simulink model "vector_control"  (R2020a)
settings: Solver=ode23t  StartTime=0.0  StopTime=2  RelTol=1e-3
libraries: powerlib x22, powerlib_meascontrol x6, simulink x4
settings Model: Creator=ahmed  LastModifiedBy=ahmed

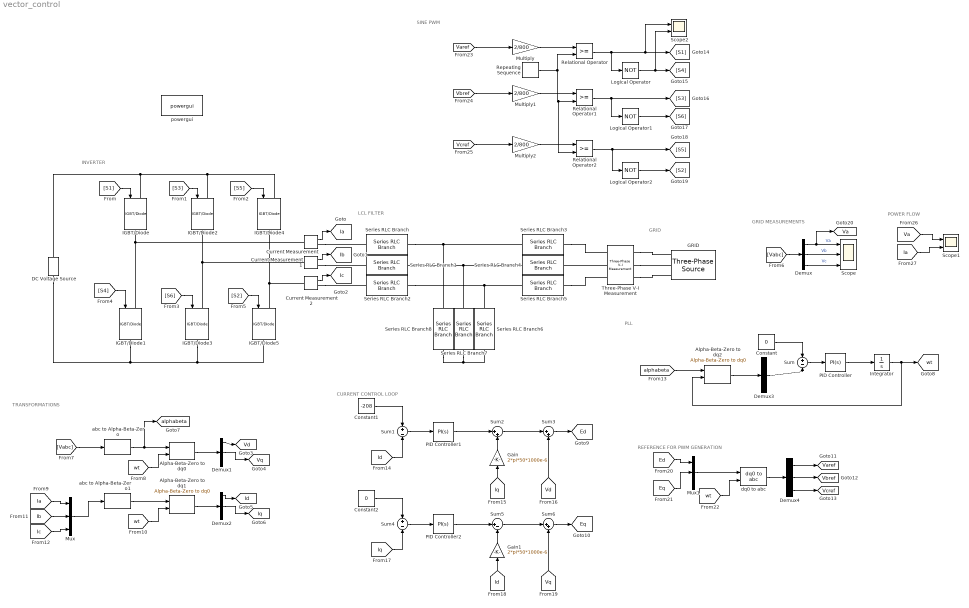
== system vector_control ==
  note: POWER FLOW
  note: GRID MEASUREMENTS
  note: GRID
  note: TRANSFORMATIONS
  note: CURRENT CONTROL LOOP
  note: REFERENCE FOR PWM GENERATION
  note: PLL
  note: SINE PWM
  note: LCL FILTER
  note: INVERTER
  Alpha-Beta-Zero to dq0 : powerlib_meascontrol/Transformations/Alpha-Beta-Zero to dq0  Alignment=90 degrees behind phase A axis
  Alpha-Beta-Zero to dq1 : powerlib_meascontrol/Transformations/Alpha-Beta-Zero to dq0  Alignment=90 degrees behind phase A axis
  Alpha-Beta-Zero to dq2 : powerlib_meascontrol/Transformations/Alpha-Beta-Zero to dq0  Alignment=90 degrees behind phase A axis
  Constant : Constant  Value=0
  Constant1 : Constant  Value=-208
  Constant2 : Constant  Value=0
  Current Measurement : powerlib/Measurements/Current Measurement  PhasorSimulation=off  OutputType=Complex  PSBequivalent=0
  Current Measurement1 : powerlib/Measurements/Current Measurement  PhasorSimulation=off  OutputType=Complex  PSBequivalent=0
  Current Measurement2 : powerlib/Measurements/Current Measurement  PhasorSimulation=off  OutputType=Complex  PSBequivalent=0
  DC Voltage Source : powerlib/Electrical Sources/DC Voltage Source  Amplitude=800  Measurements=None
  Demux{,1..4} (5 alike) : Demux  Outputs=3
  GRID : powerlib/Electrical Sources/Three-Phase Source  InternalConnection=Yg  VoltagePhases=off  Voltage=415  PhaseAngle=0  Voltage_phases=[25e3 25e3 25e3]/sqrt(3)  PhaseAngles_phases=[0 -120 +120]  Frequency=50  NonIdealSource=on  SpecifyImpedance=off  Resistance=0.001e-3  Inductance=0.001e-9  ShortCircuitLevel=100e6  BaseVoltage=415  XRratio=7  BusType=swing  Pref=10e3  Qref=0  Prefabc=[10e3, 10e3, 10e3]  Qrefabc=[0, 0, 0]  Qmin=-inf  Qmax=inf
  Gain : Gain  Gain=2*pi*50*1000e-6
  Gain1 : Gain  Gain=2*pi*50*1000e-6
  IGBT/Diode{,1..5} (6 alike) : powerlib/Power Electronics/IGBT//Diode  Ron=1e-3  Rs=1e5  Cs=inf  Measurements=off
  Integrator : Integrator
  Logical Operator : Logic  Operator=NOT  AllPortsSameDT=off  OutDataTypeStr=boolean
  Logical Operator1 : Logic  Operator=NOT  AllPortsSameDT=off  OutDataTypeStr=boolean
  Logical Operator2 : Logic  Operator=NOT  AllPortsSameDT=off  OutDataTypeStr=boolean
  Multiply : Gain  Gain=2/800
  Multiply1 : Gain  Gain=2/800
  Multiply2 : Gain  Gain=2/800
  Mux : Mux  Inputs=3
  Mux1 : Mux  Inputs=3
  PID Controller : simulink/Continuous/PID Controller  Controller=PI  Form=Parallel  TimeDomain=Continuous-time  UseExternalTs=off  SampleTime=-1  IntegratorMethod=Forward Euler  FilterMethod=Forward Euler  ControllerParametersSource=internal  P=10  I=50000  D=0  UseFilter=on  N=100  TunerSelectOption=Transfer Function Based (PID Tuner App)  InitialConditionSource=internal  InitialConditionForIntegrator=0  InitialConditionForFilter=0  DifferentiatorICPrevScaledInput=0  ExternalReset=none  TrackingMode=off  Kt=1  LimitOutput=off  UpperSaturationLimit=inf  LowerSaturationLimit=-inf  LinearizeAsGain=on  AntiWindupMode=none  Kb=1  POutMin=[]  POutMax=[]  IOutMin=[]  IOutMax=[]  DOutMin=[]  DOutMax=[]  NOutMin=[]  NOutMax=[]  SumOutMin=[]  SumOutMax=[]  SaturationOutMin=[]  SaturationOutMax=[]  PParamMin=[]  PParamMax=[]  IParamMin=[]  IParamMax=[]  DParamMin=[]  DParamMax=[]  NParamMin=[]  NParamMax=[]  KbParamMin=[]  KbParamMax=[]  KtParamMin=[]  KtParamMax=[]  KbOutMin=[]  KbOutMax=[]  KtOutMin=[]  KtOutMax=[]  IntegratorOutMin=[]  IntegratorOutMax=[]  FilterOutMin=[]  FilterOutMax=[]  SumI1OutMin=[]  SumI1OutMax=[]  SumI2OutMin=[]  SumI2OutMax=[]  SumI3OutMin=[]  SumI3OutMax=[]  SumI4OutMin=[]  SumI4OutMax=[]  SumDOutMin=[]  SumDOutMax=[]  DifferentiatorOutMin=[]  DifferentiatorOutMax=[]  FilterDiffOutCoefMin=[]  FilterDiffOutCoefMax=[]  ReciprocalOutMin=[]  ReciprocalOutMax=[]  SumDenOutMin=[]  SumDenOutMax=[]  SumNumOutMin=[]  SumNumOutMax=[]  DivideOutMin=[]  DivideOutMax=[]  UdiffTsProdOutMin=[]  UdiffTsProdOutMax=[]  NTsProdOutMin=[]  NTsProdOutMax=[]  UintegralTsProdOutMin=[]  UintegralTsProdOutMax=[]  UngainTsProdOutMin=[]  UngainTsProdOutMax=[]  IntegratorContinuousStateAttributes=''  IntegratorStateMustResolveToSignalObject=off  IntegratorRTWStateStorageClass=Auto  FilterContinuousStateAttributes=''  FilterStateMustResolveToSignalObject=off  FilterRTWStateStorageClass=Auto  ParallelPVariant=InternalParameters  IdealPVariant=Disabled  IVariant=InternalParameters  DVariant=Disabled  IntegratorVariant=Continuous  SatVariant=Disabled  AWVariant=Passthrough  PCopyVariant=Disabled  TRVariant=Disabled  FdbkBlocksVariant=Forward  IdealPFdbkVariant=Disabled  SatFdbkVariant=Disabled  DerivativeFilterVariant=Disabled  NVariant=Disabled  NCopyVariant=Disabled_SignalSpec  FilterICVariant=Disabled  IntegratorICVariant=InternalICs  ExternalResetVariant=Disabled  TRSumVariant=Passthrough  SumFdbkVariant=Disabled  SumVariant=Sum_PI  TsampFilterVariant=InternalTs  TsampNgainVariant=Passthrough  TsampIntegralVariant=Passthrough
  PID Controller1 : simulink/Continuous/PID Controller  Controller=PI  Form=Parallel  TimeDomain=Continuous-time  UseExternalTs=off  SampleTime=-1  IntegratorMethod=Forward Euler  FilterMethod=Forward Euler  ControllerParametersSource=internal  P=5  I=5000  D=0  UseFilter=on  N=100  TunerSelectOption=Transfer Function Based (PID Tuner App)  InitialConditionSource=internal  InitialConditionForIntegrator=0  InitialConditionForFilter=0  DifferentiatorICPrevScaledInput=0  ExternalReset=none  TrackingMode=off  Kt=1  LimitOutput=off  UpperSaturationLimit=inf  LowerSaturationLimit=-inf  LinearizeAsGain=on  AntiWindupMode=none  Kb=1  POutMin=[]  POutMax=[]  IOutMin=[]  IOutMax=[]  DOutMin=[]  DOutMax=[]  NOutMin=[]  NOutMax=[]  SumOutMin=[]  SumOutMax=[]  SaturationOutMin=[]  SaturationOutMax=[]  PParamMin=[]  PParamMax=[]  IParamMin=[]  IParamMax=[]  DParamMin=[]  DParamMax=[]  NParamMin=[]  NParamMax=[]  KbParamMin=[]  KbParamMax=[]  KtParamMin=[]  KtParamMax=[]  KbOutMin=[]  KbOutMax=[]  KtOutMin=[]  KtOutMax=[]  IntegratorOutMin=[]  IntegratorOutMax=[]  FilterOutMin=[]  FilterOutMax=[]  SumI1OutMin=[]  SumI1OutMax=[]  SumI2OutMin=[]  SumI2OutMax=[]  SumI3OutMin=[]  SumI3OutMax=[]  SumI4OutMin=[]  SumI4OutMax=[]  SumDOutMin=[]  SumDOutMax=[]  DifferentiatorOutMin=[]  DifferentiatorOutMax=[]  FilterDiffOutCoefMin=[]  FilterDiffOutCoefMax=[]  ReciprocalOutMin=[]  ReciprocalOutMax=[]  SumDenOutMin=[]  SumDenOutMax=[]  SumNumOutMin=[]  SumNumOutMax=[]  DivideOutMin=[]  DivideOutMax=[]  UdiffTsProdOutMin=[]  UdiffTsProdOutMax=[]  NTsProdOutMin=[]  NTsProdOutMax=[]  UintegralTsProdOutMin=[]  UintegralTsProdOutMax=[]  UngainTsProdOutMin=[]  UngainTsProdOutMax=[]  IntegratorContinuousStateAttributes=''  IntegratorStateMustResolveToSignalObject=off  IntegratorRTWStateStorageClass=Auto  FilterContinuousStateAttributes=''  FilterStateMustResolveToSignalObject=off  FilterRTWStateStorageClass=Auto  ParallelPVariant=InternalParameters  IdealPVariant=Disabled  IVariant=InternalParameters  DVariant=Disabled  IntegratorVariant=Continuous  SatVariant=Disabled  AWVariant=Passthrough  PCopyVariant=Disabled  TRVariant=Disabled  FdbkBlocksVariant=Forward  IdealPFdbkVariant=Disabled  SatFdbkVariant=Disabled  DerivativeFilterVariant=Disabled  NVariant=Disabled  NCopyVariant=Disabled_SignalSpec  FilterICVariant=Disabled  IntegratorICVariant=InternalICs  ExternalResetVariant=Disabled  TRSumVariant=Passthrough  SumFdbkVariant=Disabled  SumVariant=Sum_PI  TsampFilterVariant=InternalTs  TsampNgainVariant=Passthrough  TsampIntegralVariant=Passthrough
  PID Controller2 : simulink/Continuous/PID Controller  Controller=PI  Form=Parallel  TimeDomain=Continuous-time  UseExternalTs=off  SampleTime=-1  IntegratorMethod=Forward Euler  FilterMethod=Forward Euler  ControllerParametersSource=internal  P=5  I=5000  D=0  UseFilter=on  N=100  TunerSelectOption=Transfer Function Based (PID Tuner App)  InitialConditionSource=internal  InitialConditionForIntegrator=0  InitialConditionForFilter=0  DifferentiatorICPrevScaledInput=0  ExternalReset=none  TrackingMode=off  Kt=1  LimitOutput=off  UpperSaturationLimit=inf  LowerSaturationLimit=-inf  LinearizeAsGain=on  AntiWindupMode=none  Kb=1  POutMin=[]  POutMax=[]  IOutMin=[]  IOutMax=[]  DOutMin=[]  DOutMax=[]  NOutMin=[]  NOutMax=[]  SumOutMin=[]  SumOutMax=[]  SaturationOutMin=[]  SaturationOutMax=[]  PParamMin=[]  PParamMax=[]  IParamMin=[]  IParamMax=[]  DParamMin=[]  DParamMax=[]  NParamMin=[]  NParamMax=[]  KbParamMin=[]  KbParamMax=[]  KtParamMin=[]  KtParamMax=[]  KbOutMin=[]  KbOutMax=[]  KtOutMin=[]  KtOutMax=[]  IntegratorOutMin=[]  IntegratorOutMax=[]  FilterOutMin=[]  FilterOutMax=[]  SumI1OutMin=[]  SumI1OutMax=[]  SumI2OutMin=[]  SumI2OutMax=[]  SumI3OutMin=[]  SumI3OutMax=[]  SumI4OutMin=[]  SumI4OutMax=[]  SumDOutMin=[]  SumDOutMax=[]  DifferentiatorOutMin=[]  DifferentiatorOutMax=[]  FilterDiffOutCoefMin=[]  FilterDiffOutCoefMax=[]  ReciprocalOutMin=[]  ReciprocalOutMax=[]  SumDenOutMin=[]  SumDenOutMax=[]  SumNumOutMin=[]  SumNumOutMax=[]  DivideOutMin=[]  DivideOutMax=[]  UdiffTsProdOutMin=[]  UdiffTsProdOutMax=[]  NTsProdOutMin=[]  NTsProdOutMax=[]  UintegralTsProdOutMin=[]  UintegralTsProdOutMax=[]  UngainTsProdOutMin=[]  UngainTsProdOutMax=[]  IntegratorContinuousStateAttributes=''  IntegratorStateMustResolveToSignalObject=off  IntegratorRTWStateStorageClass=Auto  FilterContinuousStateAttributes=''  FilterStateMustResolveToSignalObject=off  FilterRTWStateStorageClass=Auto  ParallelPVariant=InternalParameters  IdealPVariant=Disabled  IVariant=InternalParameters  DVariant=Disabled  IntegratorVariant=Continuous  SatVariant=Disabled  AWVariant=Passthrough  PCopyVariant=Disabled  TRVariant=Disabled  FdbkBlocksVariant=Forward  IdealPFdbkVariant=Disabled  SatFdbkVariant=Disabled  DerivativeFilterVariant=Disabled  NVariant=Disabled  NCopyVariant=Disabled_SignalSpec  FilterICVariant=Disabled  IntegratorICVariant=InternalICs  ExternalResetVariant=Disabled  TRSumVariant=Passthrough  SumFdbkVariant=Disabled  SumVariant=Sum_PI  TsampFilterVariant=InternalTs  TsampNgainVariant=Passthrough  TsampIntegralVariant=Passthrough
  Relational Operator : RelationalOperator  OutDataTypeStr=boolean  RndMeth=Simplest
  Relational Operator1 : RelationalOperator  OutDataTypeStr=boolean  RndMeth=Simplest
  Relational Operator2 : RelationalOperator  OutDataTypeStr=boolean  RndMeth=Simplest
  Repeating Sequence : simulink/Sources/Repeating Sequence  rep_seq_t=[0 0.00005 0.0001]  rep_seq_y=[-1 1 -1]
  Scope : Scope  NumInputPorts=3
  Scope1 : Scope  NumInputPorts=2
  Scope2 : Scope  NumInputPorts=2
  Series RLC Branch{,1..5} (6 alike) : powerlib/Elements/Series RLC Branch  LConnTagsString=__new0  RConnTagsString=__new0  BranchType=L  Resistance=1  Inductance=500e-6  SetiL0=off  InitialCurrent=0  Capacitance=1e-6  Setx0=off  InitialVoltage=0  Measurements=None
  Series RLC Branch6 : powerlib/Elements/Series RLC Branch  LConnTagsString=__new0  RConnTagsString=__new0  BranchType=L  Resistance=1  Inductance=100e-6  SetiL0=off  InitialCurrent=0  Capacitance=1e-6  Setx0=off  InitialVoltage=0  Measurements=None
  Series RLC Branch7 : powerlib/Elements/Series RLC Branch  LConnTagsString=__new0  RConnTagsString=__new0  BranchType=L  Resistance=1  Inductance=100e-6  SetiL0=off  InitialCurrent=0  Capacitance=1e-6  Setx0=off  InitialVoltage=0  Measurements=None
  Series RLC Branch8 : powerlib/Elements/Series RLC Branch  LConnTagsString=__new0  RConnTagsString=__new0  BranchType=L  Resistance=1  Inductance=100e-6  SetiL0=off  InitialCurrent=0  Capacitance=1e-6  Setx0=off  InitialVoltage=0  Measurements=None
  Sum : Sum  Inputs=+-
  Sum1 : Sum  Inputs=+-
  Sum2 : Sum  Inputs=|++
  Sum3 : Sum  Inputs=|++
  Sum4 : Sum  Inputs=+-
  Sum5 : Sum  Inputs=|+-
  Sum6 : Sum  Inputs=|++
  Three-Phase V-I Measurement : powerlib/Measurements/Three-Phase V-I Measurement  VoltageMeasurement=phase-to-phase  SetLabelV=on  LabelV=Vabc  Vpu=off  VpuLL=off  CurrentMeasurement=no  SetLabelI=off  LabelI=Iabc  Ipu=off  Pbase=100e6  Vbase=500e3  OutputType=Complex  PhasorSimulation=off  PSBequivalent=0
  abc to Alpha-Beta-Zero : powerlib_meascontrol/Transformations/abc to Alpha-Beta-Zero
  abc to Alpha-Beta-Zero1 : powerlib_meascontrol/Transformations/abc to Alpha-Beta-Zero
  dq0 to abc : powerlib_meascontrol/Transformations/dq0 to abc  Alignment=90 degrees behind phase A axis
  powergui : powerlib/powergui  Priority=1  SimulationMode=Continuous  SampleTime=50e-6  frequency=60  Iterations=50  frequencyindice=50  Pbase=100e6  ErrMax=1e-4  UnitsV=kV  UnitsW=MW  buscounter=0  FunctionMessages=off  echomessages=off  EnableUseOfTLC=off  CurrentSourceSwitches=off  DisableSnubberDevices=off  DisableRonSwitches=off  DisableVfSwitches=off  DisplayEquations=off  AutomaticDiscreteSolvers=off  SolverType=Tustin/Backward Euler (TBE)  Interpol=off  ExternalGateDelay=off  methode=off  Ts=100  x0status=blocks  SPID=on  SwTol=0  HookPort=off  NonlinearTolerance=1e-4  nMaxIteration=100  ContinueOnMaxIteration=off  RestoreLinks=warning  ResistiveCurrentMeasurement=off  Frange=[0:2:500]  Ylog=off  Xlog=on  ShowGrid=off  save=off  variable=ZData  structure=0  ZoomFFT=off  StartTime=0.0  cycles=1  DisplayStyle=1  fundamental=60  FreqAxis=off  MaxFrequency=1000  frequencyindicesteady=1  RmsSteady=1  display=off
  tag scope: Ed=global, Eq=global, Ia=global, Ib=global, Ic=global, Id=global, Iq=global, Va=global, Varef=global, Vbref=global, Vcref=global, Vd=global, Vq=global, alphabeta=global, wt=global
  wires:
  [S1] -> IGBT/Diode/1
  [S3] -> IGBT/Diode2/1
  [S5] -> IGBT/Diode4/1
  [S4] -> IGBT/Diode1/1
  [S6] -> IGBT/Diode3/1
  [S2] -> IGBT/Diode5/1
  Current Measurement/1 -> [Ia]
  Current Measurement2/1 -> [Ic]
  Current Measurement1/1 -> [Ib]
  [Vabc] -> Demux/1
  Demux/2 -> Scope/2  "Vb"
  Demux/1 -> [Va], Scope/1  "Va"
  Demux/3 -> Scope/3  "Vc"
  [Vabc] -> abc to Alpha-Beta-Zero/1
  abc to Alpha-Beta-Zero/1 -> [alphabeta], Alpha-Beta-Zero to dq0/1
  [wt] -> Alpha-Beta-Zero to dq0/2
  Alpha-Beta-Zero to dq0/1 -> Demux1/1
  Demux1/1 -> [Vd]
  Demux1/2 -> [Vq]
  Demux2/2 -> [Iq]
  Demux2/1 -> [Id]
  Alpha-Beta-Zero to dq1/1 -> Demux2/1
  [wt] -> Alpha-Beta-Zero to dq1/2
  abc to Alpha-Beta-Zero1/1 -> Alpha-Beta-Zero to dq1/1
  [Ic] -> Mux/3
  [Ib] -> Mux/2
  [Ia] -> Mux/1
  Mux/1 -> abc to Alpha-Beta-Zero1/1
  [alphabeta] -> Alpha-Beta-Zero to dq2/1
  Constant/1 -> Sum/1
  Alpha-Beta-Zero to dq2/1 -> Demux3/1
  Demux3/2 -> Sum/2
  Sum/1 -> PID Controller/1
  PID Controller/1 -> Integrator/1
  Integrator/1 -> [wt], Alpha-Beta-Zero to dq2/2
  Constant1/1 -> Sum1/1
  [Id] -> Sum1/2
  Sum1/1 -> PID Controller1/1
  PID Controller1/1 -> Sum2/1
  Gain/1 -> Sum2/2
  [Iq] -> Gain/1
  [Vd] -> Sum3/2
  Sum2/1 -> Sum3/1
  Sum3/1 -> [Ed]
  Sum6/1 -> [Eq]
  Sum5/1 -> Sum6/1
  [Vq] -> Sum6/2
  [Id] -> Gain1/1
  Gain1/1 -> Sum5/2
  PID Controller2/1 -> Sum5/1
  Sum4/1 -> PID Controller2/1
  [Iq] -> Sum4/2
  Constant2/1 -> Sum4/1
  [Ed] -> Mux1/1
  [Eq] -> Mux1/2
  Mux1/1 -> dq0 to abc/1
  [wt] -> dq0 to abc/2
  dq0 to abc/1 -> Demux4/1
  Demux4/1 -> [Varef]
  Demux4/2 -> [Vbref]
  Demux4/3 -> [Vcref]
  [Varef] -> Multiply/1
  [Vbref] -> Multiply1/1
  [Vcref] -> Multiply2/1
  Multiply/1 -> Relational Operator/1
  Multiply1/1 -> Relational Operator1/1
  Multiply2/1 -> Relational Operator2/1
  Repeating Sequence/1 -> Relational Operator/2, Relational Operator2/2, Relational Operator1/2
  Relational Operator/1 -> Logical Operator/1, Scope2/1, [S1]
  Logical Operator/1 -> Scope2/2, [S4]
  Relational Operator1/1 -> Logical Operator1/1, [S3]
  Logical Operator1/1 -> [S6]
  Relational Operator2/1 -> Logical Operator2/1, [S5]
  Logical Operator2/1 -> [S2]
  [Va] -> Scope1/1
  [Ia] -> Scope1/2
  connections:
  IGBT/Diode1/LConn1 -- IGBT/Diode/RConn1 -- Current Measurement/LConn1
  IGBT/Diode3/LConn1 -- IGBT/Diode2/RConn1 -- Current Measurement1/LConn1
  IGBT/Diode5/LConn1 -- Current Measurement2/LConn1 -- IGBT/Diode4/RConn1
  IGBT/Diode/LConn1 -- DC Voltage Source/RConn1 -- IGBT/Diode2/LConn1 -- IGBT/Diode4/LConn1
  IGBT/Diode1/RConn1 -- IGBT/Diode3/RConn1 -- IGBT/Diode5/RConn1 -- DC Voltage Source/LConn1
  Series RLC Branch4/LConn1 -- Series RLC Branch7/LConn1 -- Series RLC Branch1/RConn1
  Series RLC Branch/RConn1 -- Series RLC Branch8/LConn1 -- Series RLC Branch3/LConn1
  Series RLC Branch2/RConn1 -- Series RLC Branch6/LConn1 -- Series RLC Branch5/LConn1
  Series RLC Branch8/RConn1 -- Series RLC Branch7/RConn1 -- Series RLC Branch6/RConn1
  Three-Phase V-I Measurement/LConn2 -- Series RLC Branch4/RConn1
  Series RLC Branch3/RConn1 -- Three-Phase V-I Measurement/LConn1
  Series RLC Branch5/RConn1 -- Three-Phase V-I Measurement/LConn3
  Current Measurement/RConn1 -- Series RLC Branch/LConn1
  Current Measurement1/RConn1 -- Series RLC Branch1/LConn1
  Current Measurement2/RConn1 -- Series RLC Branch2/LConn1
  Three-Phase V-I Measurement/RConn1 -- GRID/RConn1
  Three-Phase V-I Measurement/RConn2 -- GRID/RConn2
  Three-Phase V-I Measurement/RConn3 -- GRID/RConn3
